simulink model "FK_mdl"  (R2013a)
settings: Solver=ode45  StartTime=0.0  StopTime=inf  RelTol=1e-3
undefined symbols (not defined in the file or in its folder): FK, ToSimulink_Y_Signals2VRML
libraries: simulink x5, vrlib x1
settings Model: Creator=Jose Angel Rangel  LastModifiedBy=Jose Angel Rangel

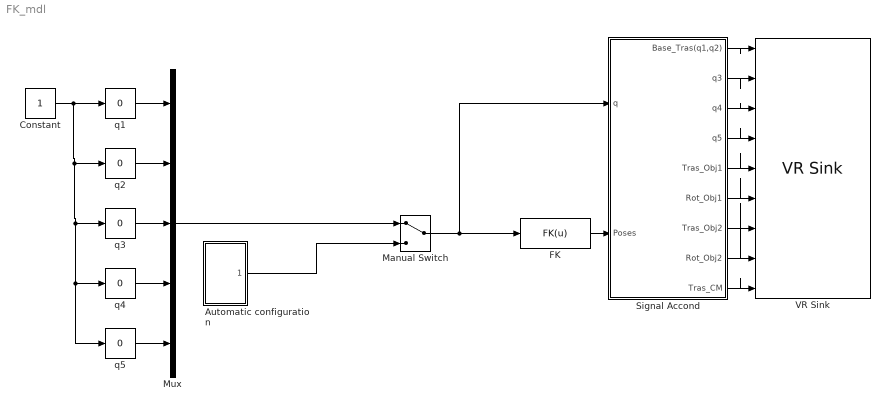
== system FK_mdl ==
  Automatic configuration : Subsystem
  Constant : Constant
  FK : MATLABFcn  MATLABFcn=FK(u)
  Manual Switch : ManualSwitch
  Mux : Mux  Inputs=5
  Signal Accond : Subsystem
  VR Sink : vrlib/VR Sink  InstantiateOnLoad=on  SampleTime=0.1  ViewEnable=on  RemoteChange=off  RemoteView=off  FieldsWritten=Base_Tras.translation.3.1.1.double#Base_Rot.rotation.4.1.1.double#Q4.rotation.4.1.1.double#Q5.rotation.4.1.1.double#Obj_RH.translation.3.1.1.double#Rot_Obj_RH.rotation.4.1.1.double#Obj_LH.translation.3.1.1.double#Rot_Obj_LH.rotation.4.1.1.double#Actual_CM.translation.3.1.1.double  WorldFileName=Simpley.wrl  AutoView=on  VideoDimensions=[]  AllowVariableSize=off  FigureProperties="{'Position', 'Name', 'Viewpoint', 'CameraBound', 'CameraDirection', 'CameraPosition', 'CameraUpVector', 'ZoomFactor', 'Antialiasing', 'Headlight', 'Lighting', 'NavPanel', 'StatusBar', 'ToolBar', 'Textures', 'Transparency', 'Triad', 'Wireframe', 'NavZones', 'NavMode', 'NavSpeed', 'CaptureFileFormat', 'CaptureFileName', 'Record2DCompressMethod', 'Record2DCompressQuality', 'Record2D', 'Record2DFileName', 'Record2DFPS'; [5.0000000000000000e+00   9.2000000000000000e+01   5.7600000000000000e+02   3.8000000000000000e+02], '', '_untitled_1', 'on', [0.0000000000000000e+00   0.0000000000000000e+00  -1.0000000000000000e+00], [0.0000000000000000e+00   0.0000000000000000e+00   0.0000000000000000e+00], [0.0000000000000000e+00   1.0000000000000000e+00   0.0000000000000000e+00], [1.0000000000000000e+00], 'on', 'on', 'on', 'halfbar', 'on', 'on', 'on', 'on', 'none', 'off', 'off', 'fly', 'normal', 'tif', '%f_anim_%n.tif', 'auto', [7.5000000000000000e+01], 'off', '%f_anim_%n.avi', [1.5000000000000000e+01]}"
  q{1..5} (5 alike) : simulink/Math Operations/Slider Gain  low=-5  gain=0  high=5
  wires:
  Constant/1 -> q5/1, q4/1, q3/1, q2/1, q1/1
  q2/1 -> Mux/2
  q3/1 -> Mux/3
  q1/1 -> Mux/1
  q4/1 -> Mux/4
  q5/1 -> Mux/5
  Mux/1 -> Manual Switch/1
  Automatic configuration/1(Auto q) -> Manual Switch/2
  Manual Switch/1 -> Signal Accond/1(q), FK/1
  FK/1 -> Signal Accond/2(Poses)
  Signal Accond/1(Base_Tras(q1,q2)) -> VR Sink/1
  Signal Accond/2(q3) -> VR Sink/2
  Signal Accond/3(q4) -> VR Sink/3
  Signal Accond/4(q5) -> VR Sink/4
  Signal Accond/5(Tras_Obj1) -> VR Sink/5
  Signal Accond/6(Rot_Obj1) -> VR Sink/6
  Signal Accond/7(Tras_Obj2) -> VR Sink/7
  Signal Accond/8(Rot_Obj2) -> VR Sink/8
  Signal Accond/9(Tras_CM) -> VR Sink/9

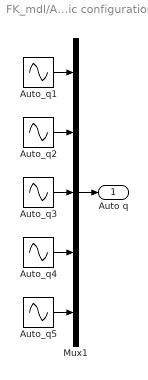
== system FK_mdl/Automatic configuration ==
  Auto_q1 : Sin  Amplitude=2*pi  Frequency=.1  SampleTime=0
  Auto_q2 : Sin  Amplitude=2*pi  Frequency=.2  SampleTime=0
  Auto_q3 : Sin  Amplitude=2*pi  Frequency=0.5  SampleTime=0
  Auto_q4 : Sin  Amplitude=2*pi  Frequency=0.8  SampleTime=0
  Auto_q5 : Sin  Amplitude=2*pi  Frequency=.3  SampleTime=0
  Mux1 : Mux  Inputs=5
  Auto q : Outport
  wires:
  Mux1/1 -> Auto q/1
  Auto_q3/1 -> Mux1/3
  Auto_q1/1 -> Mux1/1
  Auto_q5/1 -> Mux1/5
  Auto_q2/1 -> Mux1/2
  Auto_q4/1 -> Mux1/4

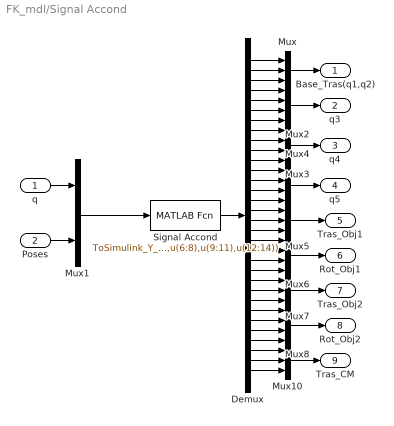
== system FK_mdl/Signal Accond ==
  q : Inport
  Poses : Inport  Port=2
  Demux : Demux  Outputs=32
  Mux{,5,7,10} (4 alike) : Mux  Inputs=3
  Mux1 : Mux  Inputs=2
  Mux{2..4,6,8} (5 alike) : Mux
  Signal Accond : MATLABFcn  MATLABFcn=ToSimulink_Y_Signals2VRML(u(1:5),u(6:8),u(9:11),u(12:14))
  Base_Tras(q1,q2) : Outport
  q3 : Outport  Port=2
  q4 : Outport  Port=3
  q5 : Outport  Port=4
  Tras_Obj1 : Outport  Port=5
  Rot_Obj1 : Outport  Port=6
  Tras_Obj2 : Outport  Port=7
  Rot_Obj2 : Outport  Port=8
  Tras_CM : Outport  Port=9
  wires:
  q/1 -> Mux1/1
  Poses/1 -> Mux1/2
  Mux1/1 -> Signal Accond/1
  Signal Accond/1 -> Demux/1
  Mux/1 -> Base_Tras(q1,q2)/1
  Mux2/1 -> q3/1
  Mux3/1 -> q4/1
  Mux4/1 -> q5/1
  Mux5/1 -> Tras_Obj1/1
  Mux6/1 -> Rot_Obj1/1
  Mux7/1 -> Tras_Obj2/1
  Mux8/1 -> Rot_Obj2/1
  Mux10/1 -> Tras_CM/1
  Demux/28 -> Mux8/3
  Demux/24 -> Mux7/2
  Demux/25 -> Mux7/3
  Demux/4 -> Mux2/1
  Demux/11 -> Mux3/4
  Demux/9 -> Mux3/2
  Demux/27 -> Mux8/2
  Demux/14 -> Mux4/3
  Demux/7 -> Mux2/4
  Demux/5 -> Mux2/2
  Demux/13 -> Mux4/2
  Demux/1 -> Mux/1
  Demux/19 -> Mux6/1
  Demux/6 -> Mux2/3
  Demux/3 -> Mux/3
  Demux/26 -> Mux8/1
  Demux/20 -> Mux6/2
  Demux/16 -> Mux5/1
  Demux/15 -> Mux4/4
  Demux/2 -> Mux/2
  Demux/21 -> Mux6/3
  Demux/23 -> Mux7/1
  Demux/10 -> Mux3/3
  Demux/12 -> Mux4/1
  Demux/22 -> Mux6/4
  Demux/18 -> Mux5/3
  Demux/17 -> Mux5/2
  Demux/29 -> Mux8/4
  Demux/8 -> Mux3/1
  Demux/32 -> Mux10/3
  Demux/31 -> Mux10/2
  Demux/30 -> Mux10/1
